simulink model "decisionTask"  (R2012b)
settings: Solver=FixedStepDiscrete  StartTime=0.0  StopTime=10.0  FixedStep=0.001  RelTol=1e-3
undefined symbols (not defined in the file or in its folder): acquireMethods, autoplayMovementDuration, autoplayReactionTime, autoplayRotationDuration, autoplayRotationStart, centerOffset, clickPercentage, clickRefractoryPeriod, clickTargetColor, clickTargetHoverColor, coherences, crossSize, cuedText, cuedTextLength, cumulativeDwell, cursorColorClick, cursorColorClosed, cursorColorOpen, cursorColors, cursorDiameter, cursorNeuralColor, cursorNonneuralColor, delayOrder, delayPeriodGainScale, displayObject, doHeadSpeedFail, drawNumbersOnTargets, dwellRefractoryPeriod, errorAssistAxis, errorAssistR, errorAssistTheta, expRandBinSize, expRandMax, expRandMin, expRandMu, eyeMode, failOnLiftoff, failurePenalty, falseClickFails, fingerPositionTolerance, fixedSeqMode, freePlayMode, gain, gloveBias, gloveLPDenominator, gloveLPNumerator, gloveNonlinearCorrection, gloveXCorrection, gloveYCorrection, gracePeriod, gridEdges, gridSize, gridTilesEachDim, headSpeedCap, holdDuration, holdTime, initialInput, initialLockout, initialState, inputType ... (+118)
(part 1 of 2)
settings Model: Creator=gilja  LastModifiedBy=NPTL
settings SolverCC: EnableConcurrentExecution=on  ConcurrentTasks=on
settings DataIOCC: SaveOutput=off  SignalLogging=off  SaveTime=off
settings OptimizationCC: InlineParams=on  InlineInvariantSignals=on  EnhancedBackFolding=on  EfficientFloat2IntCast=on  SimCompilerOptimization=On
settings DebuggingCC: UnderspecifiedInitializationDetection=Simplified
settings HardwareCC: ProdIntDivRoundTo=Zero  ProdEndianess=LittleEndian  ProdHWDeviceType=Generic->32-bit x86 compatible
settings RTWCC: SystemTargetFile=xpctarget.tlc  TemplateMakefile=xpc_default_tmf  Description=xPC Target  ProcessScript=xpctarget_make_rtw_hook  RTWCompilerOptimization=On
settings CodeAppCC: MaxIdLength=62
settings xpcTargetCC: TargetFcnLib=ansi_tfl_table_tmw.mat  CodeReplacementLibrary=XPC_BLAS  ParMdlRefBuildCompliant=on  ConcurrentExecutionCompliant=on  CombineSignalStateStructs=off  GRTInterface=on  xPCTaskExecutionProfile=on  xPCRL32EventNumber=5000  xPCisDownloadable=off  xPCLoadParamSetFile=off  xPCConcurrentTasks=off  xPCEnableSFAnimation=off

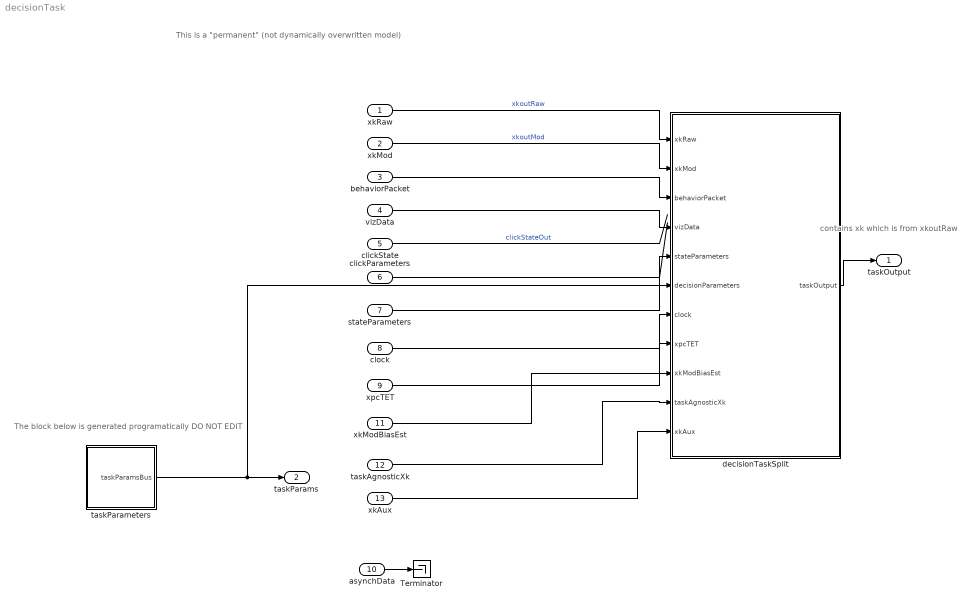
== system decisionTask ==
  note: contains xk which is
      | from xkoutRaw
  note: This is a "permanent" (not dynamically overwritten model)
  note: The block below is generated programatically
      | DO NOT EDIT
  xkRaw : Inport  OutDataTypeStr=double  PortDimensions=[double(xkConstants.NUM_STATE_DIMENSIONS),1]  SampleTime=[0.001,0]
  xkMod : Inport  Port=2  OutDataTypeStr=double  PortDimensions=[double(xkConstants.NUM_STATE_DIMENSIONS),1]  SampleTime=[0.001,0]
  behaviorPacket : Inport  Port=3  OutDataTypeStr=Bus: behaviorPacketBus  SampleTime=[0.001,0]
  vizData : Inport  Port=4  OutDataTypeStr=Bus: peripheralData  SampleTime=[0.001,0]
  clickState : Inport  Port=5  OutDataTypeStr=uint16  PortDimensions=1  SampleTime=[0.001,0]
  clickParameters : Inport  Port=6  OutDataTypeStr=Bus: clickParametersBus  SampleTime=[0.001,0]
  stateParameters : Inport  Port=7  OutDataTypeStr=Bus: stateParams  SampleTime=[0.001,0]
  clock : Inport  Port=8  OutDataTypeStr=uint32  PortDimensions=1  SampleTime=[0.001,0]
  xpcTET : Inport  Port=9  OutDataTypeStr=double  PortDimensions=1  SampleTime=[0.001,0]
  asynchData : Inport  Port=10  OutDataTypeStr=Bus: peripheralData  SampleTime=[0.001,0]
  xkModBiasEst : Inport  Port=11  OutDataTypeStr=double  PortDimensions=[double(xkConstants.NUM_STATE_DIMENSIONS),1]  SampleTime=[0.001,0]
  taskAgnosticXk : Inport  Port=12  OutDataTypeStr=double  PortDimensions=[double(xkConstants.NUM_STATE_DIMENSIONS),1]  SampleTime=[0.001,0]
  xkAux : Inport  Port=13  OutDataTypeStr=double  PortDimensions=[double(xkConstants.NUM_STATE_DIMENSIONS),1]  SampleTime=[0.001,0]
  Terminator : Terminator
  decisionTaskSplit : MATLAB Function  TreatAsAtomicUnit=on
  taskParameters : Subsystem
  taskOutput : Outport  OutDataTypeStr=Bus: taskOutput  PortDimensions=1  SampleTime=[0.001,0]  BusOutputAsStruct=on
  taskParams : Outport  Port=2  OutDataTypeStr=Bus: taskParamsBus  SampleTime=[0.001,0]
  wires:
  xkRaw/1 -> decisionTaskSplit/1(xkRaw)  "xkoutRaw"
  behaviorPacket/1 -> decisionTaskSplit/3(behaviorPacket)
  vizData/1 -> decisionTaskSplit/4(vizData)
  clickState/1 -> ?  "clickStateOut"
  clickParameters/1 -> ?
  clock/1 -> decisionTaskSplit/7(clock)
  xpcTET/1 -> decisionTaskSplit/8(xpcTET)
  stateParameters/1 -> decisionTaskSplit/5(stateParameters)
  taskParameters/1(taskParamsBus) -> taskParams/1, decisionTaskSplit/6(decisionParameters)
  decisionTaskSplit/1(taskOutput) -> taskOutput/1
  asynchData/1 -> Terminator/1
  xkMod/1 -> decisionTaskSplit/2(xkMod)  "xkoutMod"
  xkModBiasEst/1 -> decisionTaskSplit/9(xkModBiasEst)
  taskAgnosticXk/1 -> decisionTaskSplit/10(taskAgnosticXk)
  xkAux/1 -> decisionTaskSplit/11(xkAux)

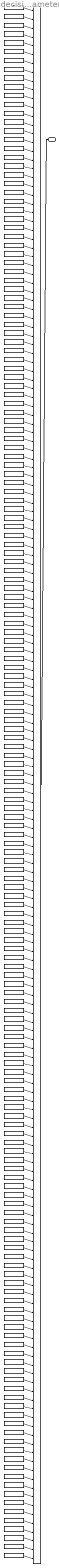
== system decisionTask/taskParameters ==
  BusOutput : BusCreator  Inputs=targetDiameter,maxTaskTime,holdTime,trialTimeout,numTrials,randomSeed,expRandMu,expRandMin,expRandMax,expRandBinSize,taskType,targetInds,numTargets,gain,failurePenalty,cursorDiameter,inputType,gloveBias,useRandomDelay,mouseOffset,workspaceX,workspaceY,workspaceZ,workspaceR,workspaceR2,showScores,trialsPerScore,cursorColorClick,recenterOnFail,recenterOnSuccess,recenterDelay,initialInput,clickPercentage,lockFingerPosition,fingerPositionTolerance,failOnLiftoff,errorAssistR,errorAssistTheta,errorAssistAxis,useGloveLPF,gloveLPNumerator,gloveLPDenominator,gloveNonlinearCorrection,gloveYCorrection,gloveXCorrection,useMouseLPF,soundOnFail,soundOnGo,soundOnSuccess,soundOnOverTarget,mouseLPNumerator,mouseLPDenominator,stopOffTarget,stopOnClick,outputType,xk2HorizontalPos,xk2HorizontalVel,xk2VerticalPos,xk2VerticalVel,xk2DepthPos,xk2DepthVel,xk2RotatePos,xk2RotateVel,xk2Rotate2Pos,xk2Rotate2Vel,gridEdges,gridTilesEachDim,selectionRefractoryMS,autoplayReactionTime,autoplayMovementDuration,powerGain,powerGainUnityCrossing,targetRotDiameter,autoplayRotationStart,autoplayRotationDuration,randomTaskTargetDiameters,randomTaskTargetRotDiameters,randomTaskBoundaries,numDisplayDims,cursorColorOpen,cursorColorClosed,showXYZaura,displayObject,preTrialLength,targetDiameters,numTargetDiameters,minTargetDistance,targetDelay,targetSpaceX,targetSpaceY,clickTargetColor,clickTargetHoverColor,falseClickFails,splitDimensions,vmrTheta,doHeadSpeedFail,headSpeedCap,eyeMode,speedTaskMode,delayPeriodGainScale,wiaMode,showWiaText,freePlayMode,drawNumbersOnTargets,xkRawSpeedCap,movementDuration,holdDuration,restDuration,returnDuration,repsPerBlock,whichMovements,movementOrder,delayOrder,textOverlayID,clickRefractoryPeriod,xpcVelocityOutputPeriodMS,outputVelocityScaling,screenUpdateRate,targetDevice,playSpokenCues,numTargetsInSeq,targetSeq,seqReadyTime,seqRehearseTime,rotateSeqCues,numRepsPerSeq,rehearsalOrder,rehearsalTimes,pathMode,memorizeMode,fixedSeqMode,sequenceMatrix,keyboard,resetDisplay,cursorNeuralColor,cursorNonneuralColor,centerOffset,scoreTime,cuedTextLength,cuedText,keyboardDims,recenterFullscreen,soundOnError,acquireMethods,cumulativeDwell,showBackspace,showStartStop,showTargetText,showTypedText,showCueOnTarget,showCueOffTarget,recenterOffset,dwellRefractoryPeriod,keyPressedTime,initialLockout,initialState,symbolMoveTimeOne,symbolRehearseTime,symbolGetReadyTime,symbolMoveTimeTwo,symbolVMRMode,symbolVMRRot,pc1MouseInControlMode,gracePeriod,maxFixDur,maxTargDur,maxStimDur,moveThresh,intertrialTime,cursorColors,gridSize,crossSize,makeGrid,tau,taskOrder,stimDur,coherences  OutDataTypeStr=Bus: taskParamsBus
  acquireMethods : Constant  Value=acquireMethods
  autoplayMovementDuration : Constant  Value=autoplayMovementDuration
  autoplayReactionTime : Constant  Value=autoplayReactionTime
  autoplayRotationDuration : Constant  Value=autoplayRotationDuration
  autoplayRotationStart : Constant  Value=autoplayRotationStart
  centerOffset : Constant  Value=centerOffset
  clickPercentage : Constant  Value=clickPercentage
  clickRefractoryPeriod : Constant  Value=clickRefractoryPeriod
  clickTargetColor : Constant  Value=clickTargetColor
  clickTargetHoverColor : Constant  Value=clickTargetHoverColor
  coherences : Constant  Value=coherences
  crossSize : Constant  Value=crossSize
  cuedText : Constant  Value=cuedText
  cuedTextLength : Constant  Value=cuedTextLength
  cumulativeDwell : Constant  Value=cumulativeDwell
  cursorColorClick : Constant  Value=cursorColorClick
  cursorColorClosed : Constant  Value=cursorColorClosed
  cursorColorOpen : Constant  Value=cursorColorOpen
  cursorColors : Constant  Value=cursorColors
  cursorDiameter : Constant  Value=cursorDiameter
  cursorNeuralColor : Constant  Value=cursorNeuralColor
  cursorNonneuralColor : Constant  Value=cursorNonneuralColor
  delayOrder : Constant  Value=delayOrder
  delayPeriodGainScale : Constant  Value=delayPeriodGainScale
  displayObject : Constant  Value=displayObject
  doHeadSpeedFail : Constant  Value=doHeadSpeedFail
  drawNumbersOnTargets : Constant  Value=drawNumbersOnTargets
  dwellRefractoryPeriod : Constant  Value=dwellRefractoryPeriod
  errorAssistAxis : Constant  Value=errorAssistAxis
  errorAssistR : Constant  Value=errorAssistR
  errorAssistTheta : Constant  Value=errorAssistTheta
  expRandBinSize : Constant  Value=expRandBinSize
  expRandMax : Constant  Value=expRandMax
  expRandMin : Constant  Value=expRandMin
  expRandMu : Constant  Value=expRandMu
  eyeMode : Constant  Value=eyeMode
  failOnLiftoff : Constant  Value=failOnLiftoff
  failurePenalty : Constant  Value=failurePenalty
  falseClickFails : Constant  Value=falseClickFails
  fingerPositionTolerance : Constant  Value=fingerPositionTolerance
  fixedSeqMode : Constant  Value=fixedSeqMode
  freePlayMode : Constant  Value=freePlayMode
  gain : Constant  Value=gain
  gloveBias : Constant  Value=gloveBias
  gloveLPDenominator : Constant  Value=gloveLPDenominator
  gloveLPNumerator : Constant  Value=gloveLPNumerator
  gloveNonlinearCorrection : Constant  Value=gloveNonlinearCorrection
  gloveXCorrection : Constant  Value=gloveXCorrection
  gloveYCorrection : Constant  Value=gloveYCorrection
  gracePeriod : Constant  Value=gracePeriod
  gridEdges : Constant  Value=gridEdges
  gridSize : Constant  Value=gridSize
  gridTilesEachDim : Constant  Value=gridTilesEachDim
  headSpeedCap : Constant  Value=headSpeedCap
  holdDuration : Constant  Value=holdDuration
  holdTime : Constant  Value=holdTime
  initialInput : Constant  Value=initialInput
  initialLockout : Constant  Value=initialLockout
  initialState : Constant  Value=initialState
  inputType : Constant  Value=inputType
  intertrialTime : Constant  Value=intertrialTime
  keyPressedTime : Constant  Value=keyPressedTime
  keyboard : Constant  Value=keyboard
  keyboardDims : Constant  Value=keyboardDims
  lockFingerPosition : Constant  Value=lockFingerPosition
  makeGrid : Constant  Value=makeGrid
  maxFixDur : Constant  Value=maxFixDur
  maxStimDur : Constant  Value=maxStimDur
  maxTargDur : Constant  Value=maxTargDur
  maxTaskTime : Constant  Value=maxTaskTime
  memorizeMode : Constant  Value=memorizeMode
  minTargetDistance : Constant  Value=minTargetDistance
  mouseLPDenominator : Constant  Value=mouseLPDenominator
  mouseLPNumerator : Constant  Value=mouseLPNumerator
  mouseOffset : Constant  Value=mouseOffset
  moveThresh : Constant  Value=moveThresh
  movementDuration : Constant  Value=movementDuration
  movementOrder : Constant  Value=movementOrder
  numDisplayDims : Constant  Value=numDisplayDims
  numRepsPerSeq : Constant  Value=numRepsPerSeq
  numTargetDiameters : Constant  Value=numTargetDiameters
  numTargets : Constant  Value=numTargets
  numTargetsInSeq : Constant  Value=numTargetsInSeq
  numTrials : Constant  Value=numTrials
  outputType : Constant  Value=outputType
  outputVelocityScaling : Constant  Value=outputVelocityScaling
  pathMode : Constant  Value=pathMode
  pc1MouseInControlMode : Constant  Value=pc1MouseInControlMode
  playSpokenCues : Constant  Value=playSpokenCues
  powerGain : Constant  Value=powerGain
  powerGainUnityCrossing : Constant  Value=powerGainUnityCrossing
  preTrialLength : Constant  Value=preTrialLength
  randomSeed : Constant  Value=randomSeed
  randomTaskBoundaries : Constant  Value=randomTaskBoundaries
  randomTaskTargetDiameters : Constant  Value=randomTaskTargetDiameters
  randomTaskTargetRotDiameters : Constant  Value=randomTaskTargetRotDiameters
  recenterDelay : Constant  Value=recenterDelay
  recenterFullscreen : Constant  Value=recenterFullscreen
  recenterOffset : Constant  Value=recenterOffset
  recenterOnFail : Constant  Value=recenterOnFail
  recenterOnSuccess : Constant  Value=recenterOnSuccess
  rehearsalOrder : Constant  Value=rehearsalOrder
  rehearsalTimes : Constant  Value=rehearsalTimes
  repsPerBlock : Constant  Value=repsPerBlock
  resetDisplay : Constant  Value=resetDisplay
  restDuration : Constant  Value=restDuration
  returnDuration : Constant  Value=returnDuration
  rotateSeqCues : Constant  Value=rotateSeqCues
  scoreTime : Constant  Value=scoreTime
  screenUpdateRate : Constant  Value=screenUpdateRate
  selectionRefractoryMS : Constant  Value=selectionRefractoryMS
  seqReadyTime : Constant  Value=seqReadyTime
  seqRehearseTime : Constant  Value=seqRehearseTime
  sequenceMatrix : Constant  Value=sequenceMatrix
  showBackspace : Constant  Value=showBackspace
  showCueOffTarget : Constant  Value=showCueOffTarget
  showCueOnTarget : Constant  Value=showCueOnTarget
  showScores : Constant  Value=showScores
  showStartStop : Constant  Value=showStartStop
  showTargetText : Constant  Value=showTargetText
  showTypedText : Constant  Value=showTypedText
  showWiaText : Constant  Value=showWiaText
  showXYZaura : Constant  Value=showXYZaura
  soundOnError : Constant  Value=soundOnError
  soundOnFail : Constant  Value=soundOnFail
  soundOnGo : Constant  Value=soundOnGo
  soundOnOverTarget : Constant  Value=soundOnOverTarget
  soundOnSuccess : Constant  Value=soundOnSuccess
  speedTaskMode : Constant  Value=speedTaskMode
  splitDimensions : Constant  Value=splitDimensions
  stimDur : Constant  Value=stimDur
  stopOffTarget : Constant  Value=stopOffTarget
  stopOnClick : Constant  Value=stopOnClick
  symbolGetReadyTime : Constant  Value=symbolGetReadyTime
  symbolMoveTimeOne : Constant  Value=symbolMoveTimeOne
  symbolMoveTimeTwo : Constant  Value=symbolMoveTimeTwo
  symbolRehearseTime : Constant  Value=symbolRehearseTime
  symbolVMRMode : Constant  Value=symbolVMRMode
  symbolVMRRot : Constant  Value=symbolVMRRot
  targetDelay : Constant  Value=targetDelay
  targetDevice : Constant  Value=targetDevice
  targetDiameter : Constant  Value=targetDiameter
  targetDiameters : Constant  Value=targetDiameters
  targetInds : Constant  Value=targetInds
  targetRotDiameter : Constant  Value=targetRotDiameter
  targetSeq : Constant  Value=targetSeq
  targetSpaceX : Constant  Value=targetSpaceX
  targetSpaceY : Constant  Value=targetSpaceY
  taskOrder : Constant  Value=taskOrder
  taskType : Constant  Value=taskType
  tau : Constant  Value=tau
  textOverlayID : Constant  Value=textOverlayID
  trialTimeout : Constant  Value=trialTimeout
  trialsPerScore : Constant  Value=trialsPerScore
  useGloveLPF : Constant  Value=useGloveLPF
  useMouseLPF : Constant  Value=useMouseLPF
  useRandomDelay : Constant  Value=useRandomDelay
  vmrTheta : Constant  Value=vmrTheta
  whichMovements : Constant  Value=whichMovements
  wiaMode : Constant  Value=wiaMode
  workspaceR : Constant  Value=workspaceR
  workspaceR2 : Constant  Value=workspaceR2
  workspaceX : Constant  Value=workspaceX
  workspaceY : Constant  Value=workspaceY
  workspaceZ : Constant  Value=workspaceZ
  xk2DepthPos : Constant  Value=xk2DepthPos
  xk2DepthVel : Constant  Value=xk2DepthVel
  xk2HorizontalPos : Constant  Value=xk2HorizontalPos
  xk2HorizontalVel : Constant  Value=xk2HorizontalVel
  xk2Rotate2Pos : Constant  Value=xk2Rotate2Pos
  xk2Rotate2Vel : Constant  Value=xk2Rotate2Vel
  xk2RotatePos : Constant  Value=xk2RotatePos
  xk2RotateVel : Constant  Value=xk2RotateVel
  xk2VerticalPos : Constant  Value=xk2VerticalPos
  xk2VerticalVel : Constant  Value=xk2VerticalVel
  xkRawSpeedCap : Constant  Value=xkRawSpeedCap
  xpcVelocityOutputPeriodMS : Constant  Value=xpcVelocityOutputPeriodMS
  taskParamsBus : Outport
  wires:
  targetDiameter/1 -> BusOutput/1  "targetDiameter"
  maxTaskTime/1 -> BusOutput/2  "maxTaskTime"
  holdTime/1 -> BusOutput/3  "holdTime"
  trialTimeout/1 -> BusOutput/4  "trialTimeout"
  numTrials/1 -> BusOutput/5  "numTrials"
  randomSeed/1 -> BusOutput/6  "randomSeed"
  expRandMu/1 -> BusOutput/7  "expRandMu"
  expRandMin/1 -> BusOutput/8  "expRandMin"
  expRandMax/1 -> BusOutput/9  "expRandMax"
  expRandBinSize/1 -> BusOutput/10  "expRandBinSize"
  taskType/1 -> BusOutput/11  "taskType"
  targetInds/1 -> BusOutput/12  "targetInds"
  numTargets/1 -> BusOutput/13  "numTargets"
  gain/1 -> BusOutput/14  "gain"
  failurePenalty/1 -> BusOutput/15  "failurePenalty"
  cursorDiameter/1 -> BusOutput/16  "cursorDiameter"
  inputType/1 -> BusOutput/17  "inputType"
  gloveBias/1 -> BusOutput/18  "gloveBias"
  useRandomDelay/1 -> BusOutput/19  "useRandomDelay"
  mouseOffset/1 -> BusOutput/20  "mouseOffset"
  workspaceX/1 -> BusOutput/21  "workspaceX"
  workspaceY/1 -> BusOutput/22  "workspaceY"
  workspaceZ/1 -> BusOutput/23  "workspaceZ"
  workspaceR/1 -> BusOutput/24  "workspaceR"
  workspaceR2/1 -> BusOutput/25  "workspaceR2"
  showScores/1 -> BusOutput/26  "showScores"
  trialsPerScore/1 -> BusOutput/27  "trialsPerScore"
  cursorColorClick/1 -> BusOutput/28  "cursorColorClick"
  recenterOnFail/1 -> BusOutput/29  "recenterOnFail"
  recenterOnSuccess/1 -> BusOutput/30  "recenterOnSuccess"
  recenterDelay/1 -> BusOutput/31  "recenterDelay"
  initialInput/1 -> BusOutput/32  "initialInput"
  clickPercentage/1 -> BusOutput/33  "clickPercentage"
  lockFingerPosition/1 -> BusOutput/34  "lockFingerPosition"
  fingerPositionTolerance/1 -> BusOutput/35  "fingerPositionTolerance"
  failOnLiftoff/1 -> BusOutput/36  "failOnLiftoff"
  errorAssistR/1 -> BusOutput/37  "errorAssistR"
  errorAssistTheta/1 -> BusOutput/38  "errorAssistTheta"
  errorAssistAxis/1 -> BusOutput/39  "errorAssistAxis"
  useGloveLPF/1 -> BusOutput/40  "useGloveLPF"
  gloveLPNumerator/1 -> BusOutput/41  "gloveLPNumerator"
  gloveLPDenominator/1 -> BusOutput/42  "gloveLPDenominator"
  gloveNonlinearCorrection/1 -> BusOutput/43  "gloveNonlinearCorrection"
  gloveYCorrection/1 -> BusOutput/44  "gloveYCorrection"
  gloveXCorrection/1 -> BusOutput/45  "gloveXCorrection"
  useMouseLPF/1 -> BusOutput/46  "useMouseLPF"
  soundOnFail/1 -> BusOutput/47  "soundOnFail"
  soundOnGo/1 -> BusOutput/48  "soundOnGo"
  soundOnSuccess/1 -> BusOutput/49  "soundOnSuccess"
  soundOnOverTarget/1 -> BusOutput/50  "soundOnOverTarget"
  mouseLPNumerator/1 -> BusOutput/51  "mouseLPNumerator"
  mouseLPDenominator/1 -> BusOutput/52  "mouseLPDenominator"
  stopOffTarget/1 -> BusOutput/53  "stopOffTarget"
  stopOnClick/1 -> BusOutput/54  "stopOnClick"
  outputType/1 -> BusOutput/55  "outputType"
  xk2HorizontalPos/1 -> BusOutput/56  "xk2HorizontalPos"
  xk2HorizontalVel/1 -> BusOutput/57  "xk2HorizontalVel"
  xk2VerticalPos/1 -> BusOutput/58  "xk2VerticalPos"
  xk2VerticalVel/1 -> BusOutput/59  "xk2VerticalVel"
  xk2DepthPos/1 -> BusOutput/60  "xk2DepthPos"
  xk2DepthVel/1 -> BusOutput/61  "xk2DepthVel"
  xk2RotatePos/1 -> BusOutput/62  "xk2RotatePos"
  xk2RotateVel/1 -> BusOutput/63  "xk2RotateVel"
  xk2Rotate2Pos/1 -> BusOutput/64  "xk2Rotate2Pos"
  xk2Rotate2Vel/1 -> BusOutput/65  "xk2Rotate2Vel"
  gridEdges/1 -> BusOutput/66  "gridEdges"
  gridTilesEachDim/1 -> BusOutput/67  "gridTilesEachDim"
  selectionRefractoryMS/1 -> BusOutput/68  "selectionRefractoryMS"
  autoplayReactionTime/1 -> BusOutput/69  "autoplayReactionTime"
  autoplayMovementDuration/1 -> BusOutput/70  "autoplayMovementDuration"
  powerGain/1 -> BusOutput/71  "powerGain"
  powerGainUnityCrossing/1 -> BusOutput/72  "powerGainUnityCrossing"
  targetRotDiameter/1 -> BusOutput/73  "targetRotDiameter"
  autoplayRotationStart/1 -> BusOutput/74  "autoplayRotationStart"
  autoplayRotationDuration/1 -> BusOutput/75  "autoplayRotationDuration"
  randomTaskTargetDiameters/1 -> BusOutput/76  "randomTaskTargetDiameters"
  randomTaskTargetRotDiameters/1 -> BusOutput/77  "randomTaskTargetRotDiameters"
  randomTaskBoundaries/1 -> BusOutput/78  "randomTaskBoundaries"
  numDisplayDims/1 -> BusOutput/79  "numDisplayDims"
  cursorColorOpen/1 -> BusOutput/80  "cursorColorOpen"
  cursorColorClosed/1 -> BusOutput/81  "cursorColorClosed"
  showXYZaura/1 -> BusOutput/82  "showXYZaura"
  displayObject/1 -> BusOutput/83  "displayObject"
  preTrialLength/1 -> BusOutput/84  "preTrialLength"
  targetDiameters/1 -> BusOutput/85  "targetDiameters"
  numTargetDiameters/1 -> BusOutput/86  "numTargetDiameters"
  minTargetDistance/1 -> BusOutput/87  "minTargetDistance"
  targetDelay/1 -> BusOutput/88  "targetDelay"
  targetSpaceX/1 -> BusOutput/89  "targetSpaceX"
  targetSpaceY/1 -> BusOutput/90  "targetSpaceY"
  clickTargetColor/1 -> BusOutput/91  "clickTargetColor"
  clickTargetHoverColor/1 -> BusOutput/92  "clickTargetHoverColor"
  falseClickFails/1 -> BusOutput/93  "falseClickFails"
  splitDimensions/1 -> BusOutput/94  "splitDimensions"
  vmrTheta/1 -> BusOutput/95  "vmrTheta"
  doHeadSpeedFail/1 -> BusOutput/96  "doHeadSpeedFail"
  headSpeedCap/1 -> BusOutput/97  "headSpeedCap"
  eyeMode/1 -> BusOutput/98  "eyeMode"
  speedTaskMode/1 -> BusOutput/99  "speedTaskMode"
  delayPeriodGainScale/1 -> BusOutput/100  "delayPeriodGainScale"
  wiaMode/1 -> BusOutput/101  "wiaMode"
  showWiaText/1 -> BusOutput/102  "showWiaText"
  freePlayMode/1 -> BusOutput/103  "freePlayMode"
  drawNumbersOnTargets/1 -> BusOutput/104  "drawNumbersOnTargets"
  xkRawSpeedCap/1 -> BusOutput/105  "xkRawSpeedCap"
  movementDuration/1 -> BusOutput/106  "movementDuration"
  holdDuration/1 -> BusOutput/107  "holdDuration"
  restDuration/1 -> BusOutput/108  "restDuration"
  returnDuration/1 -> BusOutput/109  "returnDuration"
  repsPerBlock/1 -> BusOutput/110  "repsPerBlock"
  whichMovements/1 -> BusOutput/111  "whichMovements"
  movementOrder/1 -> BusOutput/112  "movementOrder"
  delayOrder/1 -> BusOutput/113  "delayOrder"
  textOverlayID/1 -> BusOutput/114  "textOverlayID"
  clickRefractoryPeriod/1 -> BusOutput/115  "clickRefractoryPeriod"
  xpcVelocityOutputPeriodMS/1 -> BusOutput/116  "xpcVelocityOutputPeriodMS"
  outputVelocityScaling/1 -> BusOutput/117  "outputVelocityScaling"
  screenUpdateRate/1 -> BusOutput/118  "screenUpdateRate"
  targetDevice/1 -> BusOutput/119  "targetDevice"
  playSpokenCues/1 -> BusOutput/120  "playSpokenCues"
  numTargetsInSeq/1 -> BusOutput/121  "numTargetsInSeq"
  targetSeq/1 -> BusOutput/122  "targetSeq"
  seqReadyTime/1 -> BusOutput/123  "seqReadyTime"
  seqRehearseTime/1 -> BusOutput/124  "seqRehearseTime"
  rotateSeqCues/1 -> BusOutput/125  "rotateSeqCues"
  numRepsPerSeq/1 -> BusOutput/126  "numRepsPerSeq"
  rehearsalOrder/1 -> BusOutput/127  "rehearsalOrder"
  rehearsalTimes/1 -> BusOutput/128  "rehearsalTimes"
  pathMode/1 -> BusOutput/129  "pathMode"
  memorizeMode/1 -> BusOutput/130  "memorizeMode"
  fixedSeqMode/1 -> BusOutput/131  "fixedSeqMode"
  sequenceMatrix/1 -> BusOutput/132  "sequenceMatrix"
  keyboard/1 -> BusOutput/133  "keyboard"
  resetDisplay/1 -> BusOutput/134  "resetDisplay"
  cursorNeuralColor/1 -> BusOutput/135  "cursorNeuralColor"
  cursorNonneuralColor/1 -> BusOutput/136  "cursorNonneuralColor"
  centerOffset/1 -> BusOutput/137  "centerOffset"
  scoreTime/1 -> BusOutput/138  "scoreTime"
  cuedTextLength/1 -> BusOutput/139  "cuedTextLength"
  cuedText/1 -> BusOutput/140  "cuedText"
  keyboardDims/1 -> BusOutput/141  "keyboardDims"
  recenterFullscreen/1 -> BusOutput/142  "recenterFullscreen"
  soundOnError/1 -> BusOutput/143  "soundOnError"
  acquireMethods/1 -> BusOutput/144  "acquireMethods"
  cumulativeDwell/1 -> BusOutput/145  "cumulativeDwell"
  showBackspace/1 -> BusOutput/146  "showBackspace"
  showStartStop/1 -> BusOutput/147  "showStartStop"
  showTargetText/1 -> BusOutput/148  "showTargetText"
  showTypedText/1 -> BusOutput/149  "showTypedText"
  showCueOnTarget/1 -> BusOutput/150  "showCueOnTarget"
  showCueOffTarget/1 -> BusOutput/151  "showCueOffTarget"
  recenterOffset/1 -> BusOutput/152  "recenterOffset"
  dwellRefractoryPeriod/1 -> BusOutput/153  "dwellRefractoryPeriod"
  keyPressedTime/1 -> BusOutput/154  "keyPressedTime"
  initialLockout/1 -> BusOutput/155  "initialLockout"
  initialState/1 -> BusOutput/156  "initialState"
  symbolMoveTimeOne/1 -> BusOutput/157  "symbolMoveTimeOne"
  symbolRehearseTime/1 -> BusOutput/158  "symbolRehearseTime"
  symbolGetReadyTime/1 -> BusOutput/159  "symbolGetReadyTime"
  symbolMoveTimeTwo/1 -> BusOutput/160  "symbolMoveTimeTwo"
  symbolVMRMode/1 -> BusOutput/161  "symbolVMRMode"
  symbolVMRRot/1 -> BusOutput/162  "symbolVMRRot"
  pc1MouseInControlMode/1 -> BusOutput/163  "pc1MouseInControlMode"
  gracePeriod/1 -> BusOutput/164  "gracePeriod"
  maxFixDur/1 -> BusOutput/165  "maxFixDur"
  maxTargDur/1 -> BusOutput/166  "maxTargDur"
  maxStimDur/1 -> BusOutput/167  "maxStimDur"
  moveThresh/1 -> BusOutput/168  "moveThresh"
  intertrialTime/1 -> BusOutput/169  "intertrialTime"
  cursorColors/1 -> BusOutput/170  "cursorColors"
  gridSize/1 -> BusOutput/171  "gridSize"
  crossSize/1 -> BusOutput/172  "crossSize"
  makeGrid/1 -> BusOutput/173  "makeGrid"
  tau/1 -> BusOutput/174  "tau"
  taskOrder/1 -> BusOutput/175  "taskOrder"
  stimDur/1 -> BusOutput/176  "stimDur"
  coherences/1 -> BusOutput/177  "coherences"
  BusOutput/1 -> taskParamsBus/1
